simulink model "testing"  (R2016a)
settings: Solver=VariableStepAuto  StartTime=0.0  StopTime=10.0  RelTol=1e-3
undefined symbols (not defined in the file): qn
libraries: roblocks x2
settings Model: Creator=pc  LastModifiedBy=pc

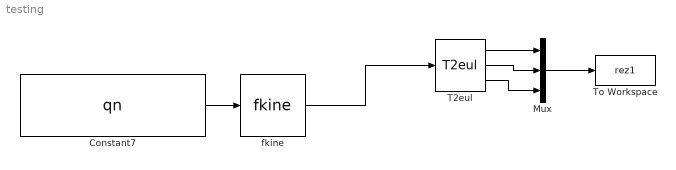
== system testing ==
  Constant7 : Constant  Value=qn
  Mux : Mux  Inputs=3
  T2eul : roblocks/Transform Conversion/T2eul
  To Workspace : ToWorkspace  VariableName=rez1  SampleTime=-1
  fkine : roblocks/Kinematics/fkine  robot=p560
  wires:
  fkine/1 -> T2eul/1
  Constant7/1 -> fkine/1
  T2eul/1 -> Mux/1
  T2eul/2 -> Mux/2
  T2eul/3 -> Mux/3
  Mux/1 -> To Workspace/1
